simulink model "Lab4"  (R2023b)
settings: Solver=ode23tb  StartTime=0  StopTime=0.04  MaxStep=1/fpwm/200  RelTol=1e-3  AbsTol=1e-3
undefined symbols (not defined in the file): Cf, fpwm, IoAVmin, Ios, Ki, Kiv, Kp, Kpv, Lf, Po, pr, ri, Rmax, Rs2, U, ucmax, Vo
libraries: spsSeriesRLCBranchLib x6, spsCurrentMeasurementLib x4, spsVoltageMeasurementLib x3, spsBreakerLib x2, spsControlledCurrentSourceLib x2, spsMeanLib x2, spsDCVoltageSourceLib x1, spsDiodeLib x1, spsMosfetLib x1, simulink x1, spspowerguiLib x1
settings Model: Creator=ist1100080  LastModifiedBy=rafae
settings SolverCC: AutoScaleAbsTol=off  AlgebraicLoopSolver=TrustRegion  MaxZcPerStep=1
settings DebuggingCC: UnconnectedInputMsg=warning  UnconnectedOutputMsg=warning  UnconnectedLineMsg=warning  SymbolicDimsDataTypeCodeGenerationDiagnostic=none
settings ModelReferenceCC: EnableRefExpFcnMdlSchedulingChecks=on
settings SFSimCC: CustomCodeUndefinedFunction=UseInterfaceOnly
settings RTWCC: DLArmComputeVersion=19.05
settings SimscapeCC: SimscapeLogType=all  SimscapeLogSimulationStatistics=on  SimscapeLogDataHistory=10000

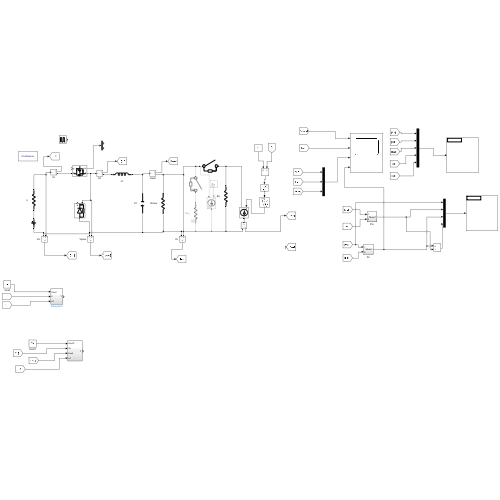
[thumbnail: Simulink's stored preview of the top-level diagram]
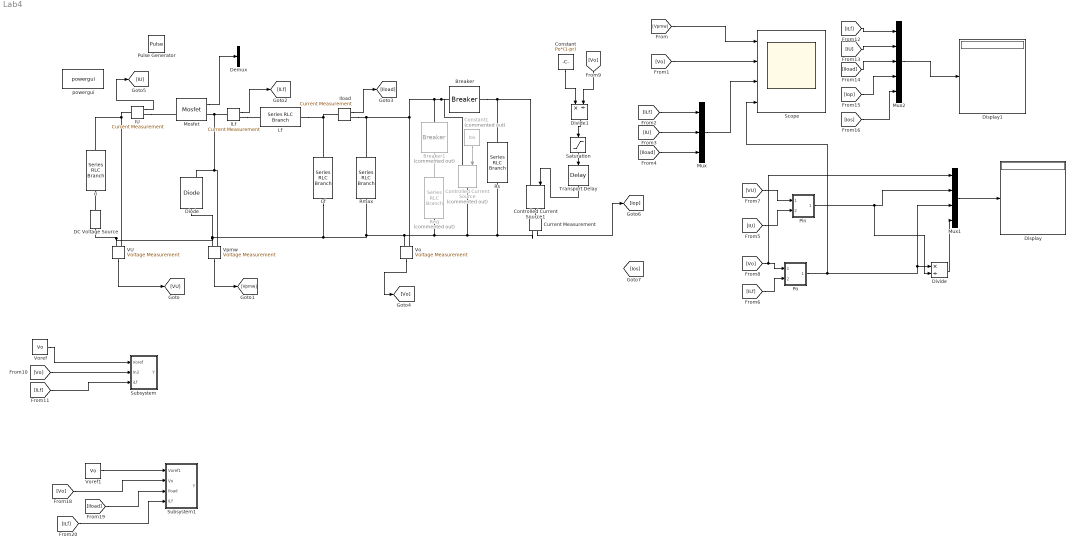
== system Lab4 ==
  Breaker : spsBreakerLib/Breaker  InitialState=0  SwitchingTimes=[0.02]  External=off  BreakerResistance=Ron  SnubberResistance=Rs  SnubberCapacitance=Cs  Measurements=None  MoreParameters=on  NoBreakLoop=off
  Breaker1 : spsBreakerLib/Breaker  Commented=on  InitialState=0  SwitchingTimes=[0.02]  External=off  BreakerResistance=Ron  SnubberResistance=Rs  SnubberCapacitance=Cs  Measurements=None  MoreParameters=on  NoBreakLoop=off
  Cf : spsSeriesRLCBranchLib/Series RLC Branch  LConnTagsString=__new0  RConnTagsString=__new0  BranchType=C  Resistance=1  Inductance=0  SetiL0=off  InitialCurrent=0  Capacitance=Cf  Setx0=on  InitialVoltage=Vo  Measurements=None
  Constant : Constant  Value=Po*(1-pr)  VectorParams1D=off
  Constant1 : Constant  Commented=on  Value=Ios
  Controlled Current Source : spsControlledCurrentSourceLib/Controlled Current Source  Commented=on  Initialize=on  Source_Type=AC  Amplitude=0  Phase=0  Frequency=0  Measurements=None
  Controlled Current Source1 : spsControlledCurrentSourceLib/Controlled Current Source  Initialize=on  Source_Type=AC  Amplitude=0  Phase=0  Frequency=0  Measurements=None
  Current Measurement : spsCurrentMeasurementLib/Current Measurement  PhasorSimulation=off  OutputType=Complex  PSBequivalent=0
  DC Voltage Source : spsDCVoltageSourceLib/DC Voltage Source  Amplitude=U  Measurements=None
  Demux : Demux  Outputs=2
  Diode : spsDiodeLib/Diode  Ron=Ron  Lon=0  Vf=Vd  IC=0  UseSnubber=0  Rs=Rs  Cs=Cs  Measurements=on
  Display : Display
  Display1 : Display
  Divide : Product  Inputs=*/
  Divide1 : Product  Inputs=*/
  ILf : spsCurrentMeasurementLib/Current Measurement  PhasorSimulation=off  OutputType=Complex  PSBequivalent=0
  IU : spsCurrentMeasurementLib/Current Measurement  PhasorSimulation=off  OutputType=Complex  PSBequivalent=0
  Iload : spsCurrentMeasurementLib/Current Measurement  PhasorSimulation=off  OutputType=Complex  PSBequivalent=0
  Lf : spsSeriesRLCBranchLib/Series RLC Branch  LConnTagsString=__new0  RConnTagsString=__new0  BranchType=L  Resistance=1  Inductance=Lf  SetiL0=off  InitialCurrent=0  Capacitance=0  Setx0=off  InitialVoltage=0  Measurements=None
  Mosfet : spsMosfetLib/Mosfet  Ron=Ron  Lon=0  Rd=Rdson  Vfd=Vd  IC=0  Rs=Rs  Cs=Cs  Measurements=on
  Mux : Mux  Inputs=3
  Mux1 : Mux
  Mux2 : Mux  Inputs=5
  Pin : Subsystem
  Po : Subsystem
  Pulse Generator : DiscretePulseGenerator  PulseType=Time based  Period=1/10000  PulseWidth=48
  Req : spsSeriesRLCBranchLib/Series RLC Branch  Commented=on  LConnTagsString=__new0  RConnTagsString=__new0  BranchType=R  Resistance=Rmax/14  Inductance=0  SetiL0=off  InitialCurrent=0  Capacitance=0  Setx0=off  InitialVoltage=0  Measurements=None
  Rmax : spsSeriesRLCBranchLib/Series RLC Branch  LConnTagsString=__new0  RConnTagsString=__new0  BranchType=R  Resistance=Vo^2/(Po*pr)  Inductance=0  SetiL0=off  InitialCurrent=0  Capacitance=0  Setx0=off  InitialVoltage=0  Measurements=None
  Rs : spsSeriesRLCBranchLib/Series RLC Branch  LConnTagsString=__new0  RConnTagsString=__new0  BranchType=R  Resistance=Rs2  Inductance=1e-3  SetiL0=off  InitialCurrent=0  Capacitance=1e-6  Setx0=off  InitialVoltage=0  Measurements=None
  Saturation : Saturate  UpperLimit=100  LowerLimit=0
  Scope : Scope  NumInputPorts=4
  Subsystem : Subsystem
  Subsystem1 : Subsystem
  Transport Delay : TransportDelay  DelayTime=1/(2*fpwm)
  VU : spsVoltageMeasurementLib/Voltage Measurement  PhasorSimulation=off  OutputType=Complex  PSBequivalent=0
  Vo : spsVoltageMeasurementLib/Voltage Measurement  PhasorSimulation=off  OutputType=Complex  PSBequivalent=0
  Voref : Constant  Value=Vo
  Voref1 : Constant  Value=Vo
  Vpmw : spsVoltageMeasurementLib/Voltage Measurement  PhasorSimulation=off  OutputType=Complex  PSBequivalent=0
  powergui : spspowerguiLib/powergui  Priority=1  SimulationMode=Continuous  SampleTime=50e-6  frequency=60  Iterations=50  frequencyindice=0  Pbase=100e6  ErrMax=1e-4  UnitsV=kV  UnitsW=MW  buscounter=0  FunctionMessages=off  echomessages=off  EnableUseOfTLC=off  CurrentSourceSwitches=off  DisableSnubberDevices=off  DisableRonSwitches=off  DisableVfSwitches=off  DisplayEquations=off  AutomaticDiscreteSolvers=off  SolverType=Tustin/Backward Euler (TBE)  Interpol=off  ExternalGateDelay=off  methode=off  Ts=100  x0status=blocks  SPID=on  SwTol=0  HookPort=off  NonlinearTolerance=1e-4  nMaxIteration=100  ContinueOnMaxIteration=off  RestoreLinks=warning  ResistiveCurrentMeasurement=off  Frange=[0:2:500]  Ylog=off  Xlog=on  ShowGrid=off  save=off  variable=ZData  structure=0  ZoomFFT=off  StartTime=0.0  cycles=1  DisplayStyle=1  fundamental=60  FreqAxis=off  MaxFrequency=1000  frequencyindicesteady=1  RmsSteady=1  display=off
  ri : spsSeriesRLCBranchLib/Series RLC Branch  LConnTagsString=__new0  RConnTagsString=__new0  BranchType=R  Resistance=ri  Inductance=0  SetiL0=off  InitialCurrent=0  Capacitance=0  Setx0=off  InitialVoltage=0  Measurements=None
  wires:
  VU/1 -> [VU]
  Vpmw/1 -> [Vpmw]
  Iload/1 -> [Iload]
  ILf/1 -> [ILf]
  Vo/1 -> [Vo]
  IU/1 -> [IU]
  Mosfet/1 -> Demux/1
  [ILf] -> Mux/1
  [IU] -> Mux/2
  [Iload] -> Mux/3
  [VU] -> Pin/1(In1)
  [IU] -> Pin/2(In2)
  Pin/1(Mean1) -> Divide/2, Mux1/2
  [Vo] -> Mux1/1, Po/1(In1)
  [ILf] -> Po/2(In2)
  Po/1(Mean1) -> Scope/4, Mux1/3, Divide/1
  Divide/1 -> Mux1/4
  Mux1/1 -> Display/1
  Mux/1 -> Scope/3
  [Vpmw] -> Scope/1
  [Vo] -> Scope/2
  [Vo] -> Divide1/2
  Constant/1 -> Divide1/1
  Divide1/1 -> Saturation/1
  Saturation/1 -> Transport Delay/1
  Transport Delay/1 -> Controlled Current Source1/1
  Constant1/1 -> Controlled Current Source/1
  Voref/1 -> Subsystem/1(Voref)
  [Vo] -> Subsystem/2(In2)
  [ILf] -> Subsystem/3(iLf)
  [Ios] -> Mux2/5
  [Iop] -> Mux2/4
  [IU] -> Mux2/2
  [Iload] -> Mux2/3
  [ILf] -> Mux2/1
  Mux2/1 -> Display1/1
  Current Measurement/1 -> [Iop]
  Voref1/1 -> Subsystem1/1(Voref1)
  [Vo] -> Subsystem1/2(Vo)
  [Iload] -> Subsystem1/3(Iload)
  [ILf] -> Subsystem1/4(iLf)
  connections:
  DC Voltage Source/RConn1 -- ri/RConn1
  ri/LConn1 -- VU/LConn1 -- IU/LConn1
  IU/RConn1 -- Mosfet/LConn1
  Mosfet/RConn1 -- Diode/RConn1 -- Vpmw/LConn1 -- ILf/LConn1
  Iload/RConn1 -- Controlled Current Source/LConn1 -- Breaker/LConn1 -- Breaker1/LConn1 -- Vo/LConn1 -- Rmax/LConn1
  ILf/RConn1 -- Lf/LConn1
  Lf/RConn1 -- Iload/LConn1 -- Cf/LConn1
  Breaker/RConn1 -- Controlled Current Source1/LConn1 -- Rs/LConn1
  Req/LConn1 -- Breaker1/RConn1
  VU/LConn2 -- Diode/LConn1 -- Cf/RConn1 -- Current Measurement/RConn1 -- Rs/RConn1 -- Controlled Current Source/RConn1 -- Req/RConn1 -- Vo/LConn2 -- Rmax/RConn1 -- Vpmw/LConn2 -- DC Voltage Source/LConn1
  Controlled Current Source1/RConn1 -- Current Measurement/LConn1

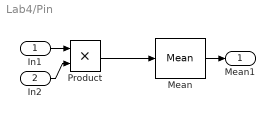
== system Lab4/Pin ==
  In1 : Inport
  In2 : Inport  Port=2
  Mean : spsMeanLib/Mean  Freq=0.1*fpwm  Vinit=110  Ts=0
  Product : Product
  Mean1 : Outport
  wires:
  Product/1 -> Mean/1
  In2/1 -> Product/2
  In1/1 -> Product/1
  Mean/1 -> Mean1/1

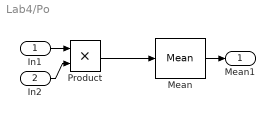
== system Lab4/Po ==
  In1 : Inport
  In2 : Inport  Port=2
  Mean : spsMeanLib/Mean  Freq=0.1*fpwm  Vinit=110  Ts=0
  Product : Product
  Mean1 : Outport
  wires:
  Product/1 -> Mean/1
  In2/1 -> Product/2
  In1/1 -> Product/1
  Mean/1 -> Mean1/1

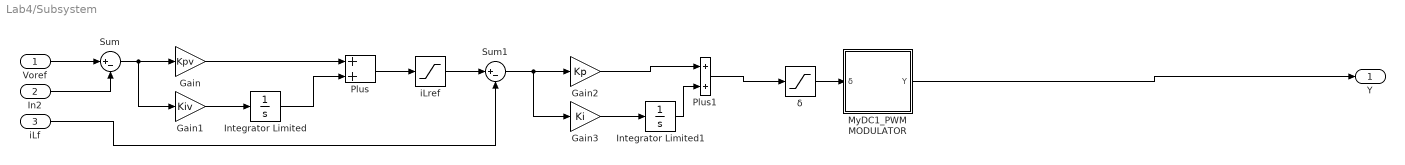
== system Lab4/Subsystem ==
  Voref : Inport
  In2 : Inport  Port=2
  iLf : Inport  Port=3
  Gain : Gain  Gain=Kpv
  Gain1 : Gain  Gain=Kiv
  Gain2 : Gain  Gain=Kp
  Gain3 : Gain  Gain=Ki
  Integrator Limited : Integrator  LimitOutput=on  UpperSaturationLimit=60  LowerSaturationLimit=-60
  Integrator Limited1 : Integrator  LimitOutput=on  UpperSaturationLimit=1  LowerSaturationLimit=-1
  MyDC1_PWM MODULATOR : Subsystem
  Plus : Sum
  Plus1 : Sum
  Sum : Sum  Inputs=|+-
  Sum1 : Sum  Inputs=|+-
  iLref : Saturate  UpperLimit=60  LowerLimit=0
  δ : Saturate  UpperLimit=0.99  LowerLimit=0.01
  Y : Outport
  wires:
  Plus1/1 -> δ/1
  Gain3/1 -> Integrator Limited1/1
  Voref/1 -> Sum/1
  Sum1/1 -> Gain3/1, Gain2/1
  Gain1/1 -> Integrator Limited/1
  Sum/1 -> Gain1/1, Gain/1
  iLf/1 -> Sum1/2
  In2/1 -> Sum/2
  Integrator Limited/1 -> Plus/2
  Gain/1 -> Plus/1
  Gain2/1 -> Plus1/1
  δ/1 -> MyDC1_PWM MODULATOR/1(δ)
  Integrator Limited1/1 -> Plus1/2
  iLref/1 -> Sum1/1
  Plus/1 -> iLref/1
  MyDC1_PWM MODULATOR/1(Y) -> Y/1

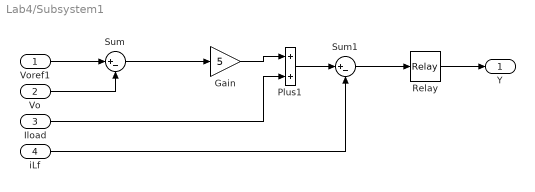
== system Lab4/Subsystem1 ==
  Voref1 : Inport
  Vo : Inport  Port=2
  Iload : Inport  Port=3
  iLf : Inport  Port=4
  Gain : Gain  Gain=5
  Plus1 : Sum
  Relay : Relay  OnSwitchValue=IoAVmin/2  OffSwitchValue=-IoAVmin/2
  Sum : Sum  Inputs=|+-
  Sum1 : Sum  Inputs=|+-
  Y : Outport
  wires:
  Vo/1 -> Sum/2
  Sum/1 -> Gain/1
  Relay/1 -> Y/1
  Plus1/1 -> Sum1/1
  iLf/1 -> Sum1/2
  Sum1/1 -> Relay/1
  Gain/1 -> Plus1/1
  Voref1/1 -> Sum/1
  Iload/1 -> Plus1/2

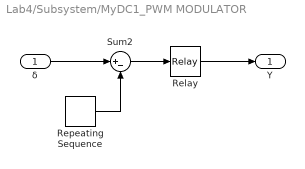
== system Lab4/Subsystem/MyDC1_PWM MODULATOR ==
  δ : Inport
  Relay : Relay  OnSwitchValue=0.01  OffSwitchValue=-0.01
  Repeating Sequence : simulink/Sources/Repeating Sequence  rep_seq_t=[0 1/fpwm]  rep_seq_y=[0 ucmax]
  Sum2 : Sum  Inputs=|+-
  Y : Outport
  wires:
  Repeating Sequence/1 -> Sum2/2
  δ/1 -> Sum2/1
  Sum2/1 -> Relay/1
  Relay/1 -> Y/1
